simulink model "Up_Wait_Down"  (R2025b)
settings: Solver=FixedStepDiscrete  StartTime=0.0  StopTime=10.0  FixedStep=0.01  RelTol=1e-3
settings Model: Creator=soura  LastModifiedBy=soura

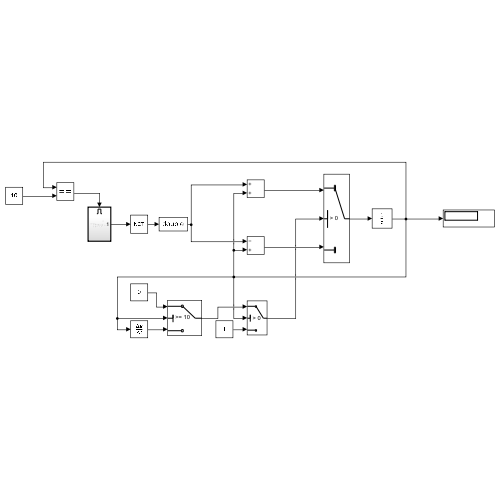
[thumbnail: Simulink's stored preview of the top-level diagram]
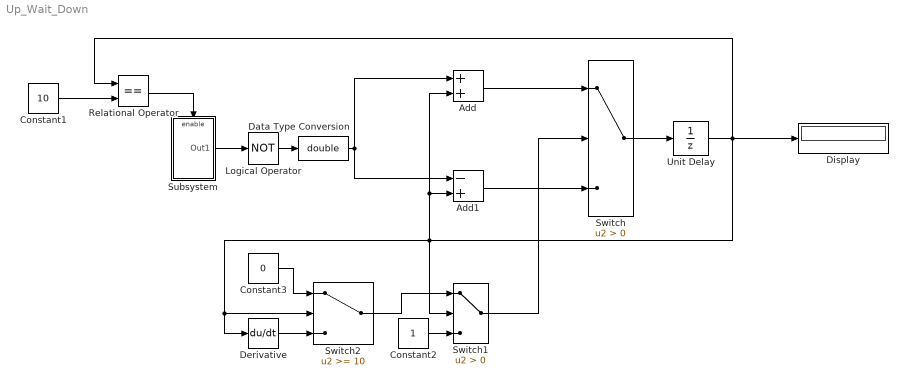
== system Up_Wait_Down ==
  Add : Sum
  Add1 : Sum  Inputs=-+
  Constant1 : Constant  Value=10
  Constant2 : Constant
  Constant3 : Constant  Value=0
  Data Type Conversion : DataTypeConversion  OutDataTypeStr=double  SaturateOnIntegerOverflow=off  RndMeth=Floor
  Derivative : Derivative
  Display : Display
  Logical Operator : Logic  Operator=NOT  AllPortsSameDT=off  OutDataTypeStr=boolean
  Relational Operator : RelationalOperator  Operator===  OutDataTypeStr=boolean  RndMeth=Simplest  InputSameDT=off
  Subsystem : Subsystem
  Switch : Switch  Criteria=u2 > Threshold  SaturateOnIntegerOverflow=off  InputSameDT=off
  Switch1 : Switch  Criteria=u2 > Threshold  SaturateOnIntegerOverflow=off  InputSameDT=off
  Switch2 : Switch  Threshold=10  SaturateOnIntegerOverflow=off  InputSameDT=off
  Unit Delay : UnitDelay  SampleTime=-1  HasFrameUpgradeWarning=on
  wires:
  Constant2/1 -> Switch1/3
  Add/1 -> Switch/1
  Derivative/1 -> Switch2/3
  Add1/1 -> Switch/3
  Logical Operator/1 -> Data Type Conversion/1
  Switch/1 -> Unit Delay/1
  Constant1/1 -> Relational Operator/2
  Switch2/1 -> Switch1/1
  Relational Operator/1 -> Subsystem/Enable
  Constant3/1 -> Switch2/1
  Data Type Conversion/1 -> Add/1, Add1/1
  Unit Delay/1 -> Relational Operator/1, Display/1, Switch1/2, Derivative/1, Switch2/2, Add/2, Add1/2
  Subsystem/1(Out1) -> Logical Operator/1
  Switch1/1 -> Switch/2

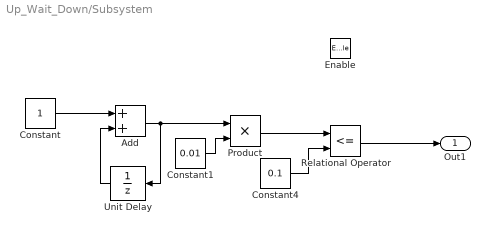
== system Up_Wait_Down/Subsystem ==
  Enable : EnablePort
  Add : Sum
  Constant : Constant
  Constant1 : Constant  Value=0.01
  Constant4 : Constant  Value=0.1
  Product : Product
  Relational Operator : RelationalOperator  Operator=<=  OutDataTypeStr=boolean  RndMeth=Simplest  InputSameDT=off
  Unit Delay : UnitDelay  SampleTime=-1  HasFrameUpgradeWarning=on
  Out1 : Outport  OutputWhenDisabled=reset  InitialOutput=0
  wires:
  Relational Operator/1 -> Out1/1
  Constant4/1 -> Relational Operator/2
  Product/1 -> Relational Operator/1
  Unit Delay/1 -> Add/2
  Constant/1 -> Add/1
  Add/1 -> Product/1, Unit Delay/1
  Constant1/1 -> Product/2
